simulink model "AdaptiveThresholdLocalMaxima"  (R2020a)
settings: Solver=VariableStepAuto  StartTime=0.0  StopTime=10  RelTol=1e-3
libraries: simulink x2, sdolib x1, dspswit3 x1, dspfdesign x1, dspstat3 x1, hdlsllib x1
settings Model: Creator=sbuccelli  LastModifiedBy=diflo

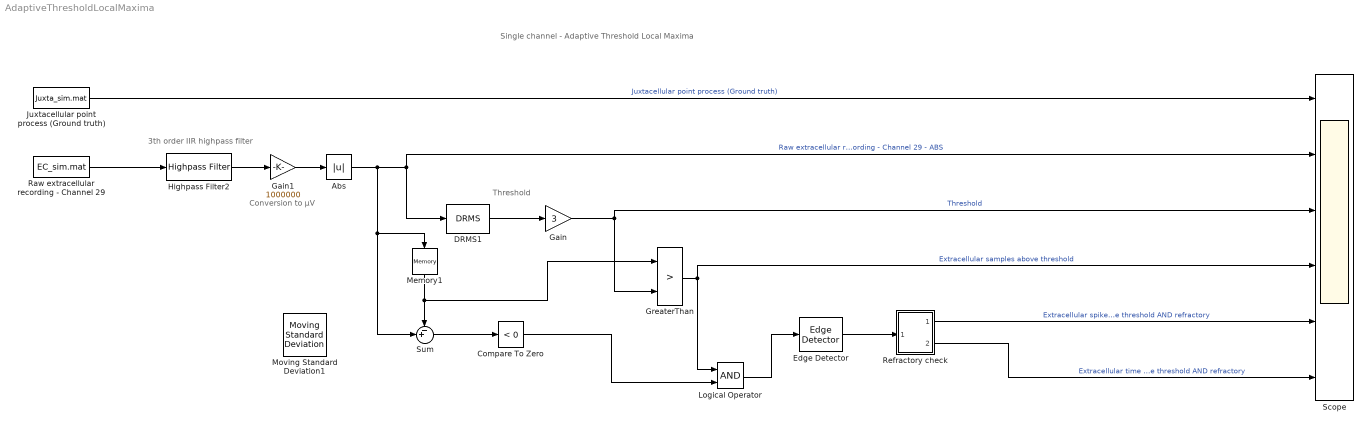
== system AdaptiveThresholdLocalMaxima ==
  note: Threshold
  note: Conversion to μV
  note: 3th order IIR highpass filter
  note: Single channel - Adaptive Threshold Local Maxima
  Abs : Abs
  Compare To Zero : simulink/Logic and Bit Operations/Compare To Zero  relop=<  OutDataTypeStr=boolean
  DRMS1 : sdolib/RMS Blocks/DRMS  Ts=1/30000
      settings: SourceProductBaseCode=SO
  Edge Detector : dspswit3/Edge Detector  InputProcessing=Columns as channels (frame based)
      settings: SourceProductBaseCode=DS
  Gain : Gain  Gain=3
  Gain1 : Gain  Gain=1000000
  GreaterThan : RelationalOperator  Operator=>  OutDataTypeStr=boolean  RndMeth=Simplest
  Highpass Filter2 : dspfdesign/Highpass Filter  FilterType=IIR  DesignForMinimumOrder=off  FilterOrder=3  StopbandFrequency=1  PassbandFrequency=300  StopbandAttenuation=80  PassbandRipple=0.1  InheritSampleRate=off  SampleRate=30000  SimulateUsing=Interpreted execution  roundingMode=Floor  coeffsDataTypeStr=fixdt(1,16)
  Juxtacellular point process (Ground truth) : FromFile  FileName=Juxta_sim.mat  SampleTime=1/30000
  Logical Operator : Logic  AllPortsSameDT=off  OutDataTypeStr=boolean
  Memory1 : Memory  InheritSampleTime=on
  Moving Standard Deviation1 : dspstat3/Moving Standard Deviation  Method=Sliding window  ForgettingFactorPort=off  SpecifyWindowLength=on  WindowLength=30000  ForgettingFactor=0.9  SimulateUsing=Code generation
      settings: SourceProductBaseCode=DS
  Raw extracellular recording - Channel 29 : FromFile  FileName=EC_sim.mat  SampleTime=1/30000
  Refractory check : Subsystem
  Scope : Scope  NumInputPorts=6
  Sum : Sum  Inputs=-+|
  wires:
  Juxtacellular point process (Ground truth)/1 -> Scope/1  "Juxtacellular point process (Ground truth)"
  Raw extracellular recording - Channel 29/1 -> Highpass Filter2/1
  Edge Detector/1 -> Refractory check/1("   ")
  Refractory check/2(Output) -> Scope/6  "Extracellular time since last spike above threshold AND refractory"
  GreaterThan/1 -> Logical Operator/1, Scope/4  "Extracellular samples above threshold"
  Gain/1 -> GreaterThan/2, Scope/3  "Threshold"
  DRMS1/1 -> Gain/1
  Highpass Filter2/1 -> Gain1/1
  Refractory check/1(" ") -> Scope/5  "Extracellular spikes above threshold AND refractory"
  Gain1/1 -> Abs/1
  Memory1/1 -> GreaterThan/1, Sum/1
  Compare To Zero/1 -> Logical Operator/2
  Logical Operator/1 -> Edge Detector/1
  Sum/1 -> Compare To Zero/1
  Abs/1 -> Sum/2, Memory1/1, Scope/2, DRMS1/1  "Raw extracellular recording - Channel 29 - ABS"

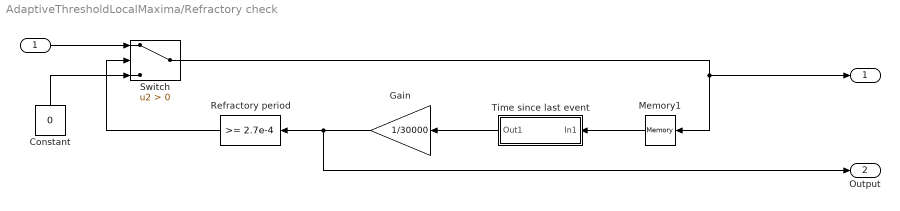
== system AdaptiveThresholdLocalMaxima/Refractory check ==
  "   " : Inport
  Constant : Constant  Value=0
  Gain : Gain  Gain=1/30000  ParamDataTypeStr=double
  Memory1 : Memory  InheritSampleTime=on
  Refractory period : simulink/Logic and Bit Operations/Compare To Constant  relop=>=  const=2.7e-4  OutDataTypeStr=boolean
  Switch : Switch  Criteria=u2 > Threshold
  Time since last event : Subsystem
  " " : Outport
  Output : Outport  Port=2
  wires:
  "   "/1 -> Switch/1
  Memory1/1 -> Time since last event/1(In1)
  Time since last event/1(Out1) -> Gain/1
  Constant/1 -> Switch/3
  Gain/1 -> Refractory period/1, Output/1
  Switch/1 -> " "/1, Memory1/1
  Refractory period/1 -> Switch/2

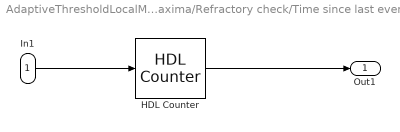
== system AdaptiveThresholdLocalMaxima/Refractory check/Time since last event ==
  In1 : Inport
  HDL Counter : hdlsllib/Sources/HDL Counter  CountType=Free running  CountInit=1  CountStep=1  CountMax=25  CountFromType=Initial value  CountFrom=1  CountResetPort=on  CountLoadPort=off  CountEnbPort=off  CountDirPort=off  CountDataType=Unsigned  CountWordLen=32  CountFracLen=0  CountSampTime=1
  Out1 : Outport
  wires:
  In1/1 -> HDL Counter/1
  HDL Counter/1 -> Out1/1
